simulink library "Battery"  (R2021a)
settings: Solver=VariableStepAuto  StartTime=0.0  StopTime=10.0  RelTol=1e-3
settings Model: Creator=yavuz  LastModifiedBy=yavuz

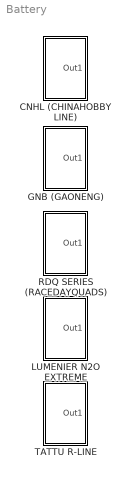
== system Battery ==
  CNHL (CHINAHOBBYLINE) : Subsystem
  GNB (GAONENG) : Subsystem
  LUMENIER N2O EXTREME : Subsystem
  RDQ SERIES (RACEDAYQUADS) : Subsystem
  TATTU R-LINE : Subsystem

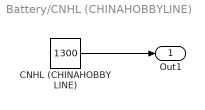
== system Battery/CNHL (CHINAHOBBYLINE) ==
  CNHL (CHINAHOBBYLINE) : Constant  Value=1300
  Out1 : Outport
  wires:
  CNHL (CHINAHOBBYLINE)/1 -> Out1/1

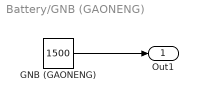
== system Battery/GNB (GAONENG) ==
  GNB (GAONENG) : Constant  Value=1500
  Out1 : Outport
  wires:
  GNB (GAONENG)/1 -> Out1/1

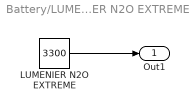
== system Battery/LUMENIER N2O EXTREME ==
  LUMENIER N2O EXTREME : Constant  Value=3300
  Out1 : Outport
  wires:
  LUMENIER N2O EXTREME/1 -> Out1/1

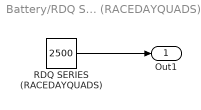
== system Battery/RDQ SERIES (RACEDAYQUADS) ==
  RDQ SERIES (RACEDAYQUADS) : Constant  Value=2500
  Out1 : Outport
  wires:
  RDQ SERIES (RACEDAYQUADS)/1 -> Out1/1

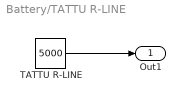
== system Battery/TATTU R-LINE ==
  TATTU R-LINE : Constant  Value=5000
  Out1 : Outport
  wires:
  TATTU R-LINE/1 -> Out1/1
